simulink library "DataTypePropCastLib"  (R2019b)
settings: Solver=VariableStepAuto  StartTime=0.0  StopTime=10.0  RelTol=1e-3
undefined symbols (not defined in the file): NumBits1, NumBits2
libraries: $bdroot x2, simulink x2
settings Model: Creator=edenaxas  LastModifiedBy=andyb

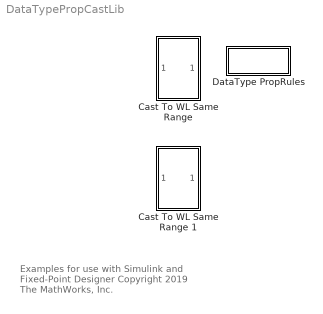
== system DataTypePropCastLib ==
  note: Examples for use with
      | Simulink and Fixed-Point Designer
      | Copyright 2019 The MathWorks, Inc.
  "Cast To WL Same Range " : Subsystem  mask(Cast to WL Same Range){CastWL=16}
      mask prompts: CastWL "Word Length"
      mask help: Cast to a specific word length while maintaining the range
      mask Display: fprintf('WL=%d', CastWL)
  Cast To WL Same Range 1 : Subsystem  mask(Cast to WL Same Range){CastWL=16}
      mask prompts: CastWL "Word Length"
      mask help: Cast to a specific word length while maintaining the range
      mask Display: fprintf('WL=%d', CastWL)
  DataType PropRules : Subsystem
      mask Display: fprintf('Data Type\nProp Rules')

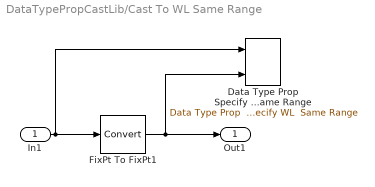
== system DataTypePropCastLib/Cast To WL Same Range  ==
  In1 : Inport
  Data Type Prop Specify WL Same Range : $bdroot/Data Type Prop  Specify WL  Same Range  WLParam=CastWL
  FixPt To FixPt1 : DataTypeConversion  SaturateOnIntegerOverflow=on
  Out1 : Outport
  wires:
  In1/1 -> FixPt To FixPt1/1, Data Type Prop Specify WL Same Range/1
  FixPt To FixPt1/1 -> Data Type Prop Specify WL Same Range/2, Out1/1

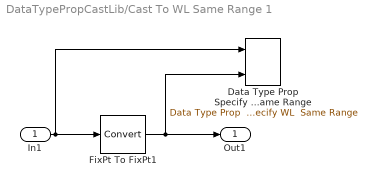
== system DataTypePropCastLib/Cast To WL Same Range 1 ==
  In1 : Inport
  Data Type Prop Specify WL Same Range : $bdroot/Data Type Prop  Specify WL  Same Range  WLParam=CastWL
  FixPt To FixPt1 : DataTypeConversion  SaturateOnIntegerOverflow=on
  Out1 : Outport
  wires:
  FixPt To FixPt1/1 -> Out1/1, Data Type Prop Specify WL Same Range/2
  In1/1 -> Data Type Prop Specify WL Same Range/1, FixPt To FixPt1/1

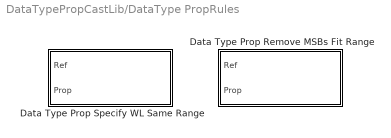
== system DataTypePropCastLib/DataType PropRules ==
  Data Type Prop Remove MSBs Fit Range : Subsystem  mask(Data Type Prop Keep Specified MSBs){designVals=16}
      mask prompts: designVals "Design Values Vector"
      mask help:
      | Based on the reference port data type, set the prop port data type to have the same most significant bit (MSB) locations, but a limited word length.
      |
      | For integer and fixed-point, the propagated port will have the same data type as the reference port except that some
      | least significant bits (LSBs) may be removed. LSBs will be removed if Max Prop Port Word Length parameter is smaller than the reference port word length.
      | The prop port word length obeys this formula
      |     propWL = min( MaxPropWL, refWL )
      |
      | If the reference port is floating point, then the propagated port will also be floating point.
      |
      | Note: the prop port data type has the same range as the reference port data type in the following sense.
      | If a signal with reference port data type is cast to the prop port data type with rounding mode set to floor or simplest, then the cast will never overflow.
      | Input values can be slightly larger than the maximum representable output value, but round to floor or simplest will set the extra LSBs to zero and reduce the value to be in range of the output.
      mask init:
      | minDesignVal = min(designVals);
      | maxDesignVal = max(designVals);
      mask Display: fprintf('Propagate\nRemove MSBs\nFit Range\n[%g..%g]',minDesignVal,maxDesignVal)
  Data Type Prop Specify WL Same Range : Subsystem  mask(Data Type Prop Keep Specified MSBs){WLParam=16}
      mask prompts: WLParam "Max Prop Port Word Length"
      mask help:
      | Based on the reference port data type, set the prop port data type to have the same most significant bit (MSB) locations, but a limited word length.
      |
      | For integer and fixed-point, the propagated port will have the same data type as the reference port except that some
      | least significant bits (LSBs) may be removed. LSBs will be removed if Max Prop Port Word Length parameter is smaller than the reference port word length.
      | The prop port word length obeys this formula
      |     propWL = min( MaxPropWL, refWL )
      |
      | If the reference port is floating point, then the propagated port will also be floating point.
      |
      | Note: the prop port data type has the same range as the reference port data type in the following sense.
      | If a signal with reference port data type is cast to the prop port data type with rounding mode set to floor or simplest, then the cast will never overflow.
      | Input values can be slightly larger than the maximum representable output value, but round to floor or simplest will set the extra LSBs to zero and reduce the value to be in range of the output.
      mask Display: fprintf('Propagate\nKeep MSB\npropWL=\nmin(%d,refWL)', WLParam)

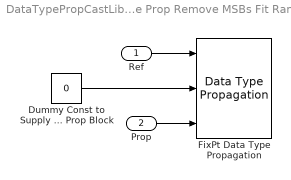
== system DataTypePropCastLib/DataType PropRules/Data Type Prop Remove MSBs Fit Range ==
  Ref : Inport
  Prop : Inport  Port=2
  Dummy Const to Supply Data Type to Prop Block : Constant  Value=0  OutDataTypeStr=fixdt(0,WLParam,0)
  FixPt Data Type Propagation : simulink/Signal Attributes/Data Type Propagation  PropDataType=sfix(16)  IfRefDouble=double  IfRefSingle=single  IsSigned=IsSigned1  NumBitsBase=min([NumBits1 NumBits2])  NumBitsMult=1  NumBitsAdd=0  NumBitsAllowFinal=1:128  PropScaling=2^-10  ValuesUsedBestPrec=[5 -7]  SlopeBase=PosRange1  SlopeMult=1  SlopeAdd=0  BiasBase=Bias1  BiasMult=1  BiasAdd=0
      settings: SourceProductBaseCode=SL
  wires:
  Dummy Const to Supply Data Type to Prop Block/1 -> FixPt Data Type Propagation/2
  Prop/1 -> FixPt Data Type Propagation/3
  Ref/1 -> FixPt Data Type Propagation/1

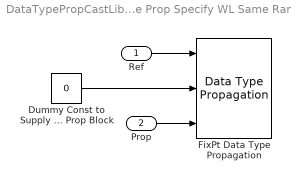
== system DataTypePropCastLib/DataType PropRules/Data Type Prop Specify WL Same Range ==
  Ref : Inport
  Prop : Inport  Port=2
  Dummy Const to Supply Data Type to Prop Block : Constant  Value=0  OutDataTypeStr=fixdt(0,WLParam,0)
  FixPt Data Type Propagation : simulink/Signal Attributes/Data Type Propagation  PropDataType=sfix(16)  IfRefDouble=double  IfRefSingle=single  IsSigned=IsSigned1  NumBitsBase=min([NumBits1 NumBits2])  NumBitsMult=1  NumBitsAdd=0  NumBitsAllowFinal=1:128  PropScaling=2^-10  ValuesUsedBestPrec=[5 -7]  SlopeBase=PosRange1  SlopeMult=1  SlopeAdd=0  BiasBase=Bias1  BiasMult=1  BiasAdd=0
      settings: SourceProductBaseCode=SL
  wires:
  Ref/1 -> FixPt Data Type Propagation/1
  Prop/1 -> FixPt Data Type Propagation/3
  Dummy Const to Supply Data Type to Prop Block/1 -> FixPt Data Type Propagation/2
